simulink model "groundStation001_th"  (R2018b)
settings: Solver=VariableStepAuto  StartTime=0.0  StopTime=sim_time  FixedStep=1e-2  MaxStep=.1  RelTol=1e-3
values from neighbouring files (symbols this model uses):
  initPos = [0 0 100]    [groundStation001_ts.m]    (also in groundStation001_ts2.m)
  objectHeight = platformVolume^(1/3)    (= 1.51829448594)    [groundStation001_ts.m]    (also in groundStation001_ts2.m)
  platformInertiaMatrix = ((1/6)*platformMass*objectHeight^2).*eye(3)    [groundStation001_ts.m]    (also in groundStation001_ts2.m = ((1/6)*platformMass*platformVolume^(2/3)).*eye(3))
  thrs = OCT.tethers    [groundStation001_ts2.m]
libraries: vectorNormalizer_ul x1, constantUniformFlow_ul x1, groundStation001_cl x1
settings Model: Creator=Erin B  LastModifiedBy=Erin B

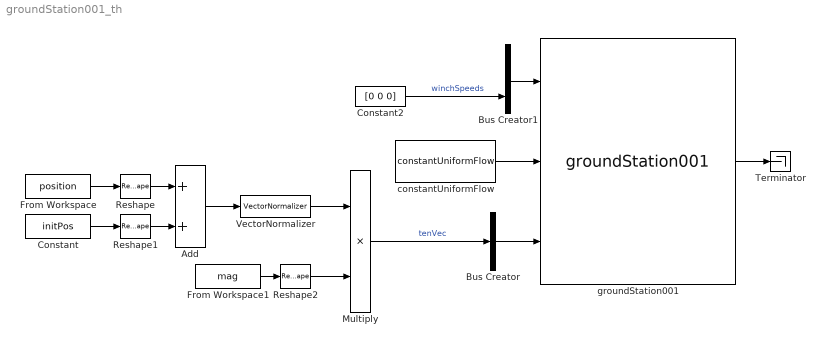
== system groundStation001_th ==
  Add : Sum
  Bus Creator : BusCreator  Inputs=1  OutDataTypeStr=Bus: thrTenVecBus  NonVirtualBus=on
  Bus Creator1 : BusCreator  Inputs=2  OutDataTypeStr=Bus: ctrlBus  NonVirtualBus=on
  Constant : Constant  Value=initPos
  Constant2 : Constant  Value=[0 0 0]
  From Workspace : FromWorkspace  VariableName=position  SampleTime=0
  From Workspace1 : FromWorkspace  VariableName=mag  SampleTime=0
  Multiply : Product
  Reshape : Reshape  OutputDimensionality=Column vector (2-D)
  Reshape1 : Reshape  OutputDimensionality=Column vector (2-D)
  Reshape2 : Reshape  OutputDimensionality=Column vector (2-D)
  Terminator : Terminator
  "VectorNormalizer " : vectorNormalizer_ul/VectorNormalizer   SystemSampleTime=-1
  constantUniformFlow : constantUniformFlow_ul/constantUniformFlow  SystemSampleTime=-1  VariantControl=VSS_environment_constantUniformFlow
  groundStation001 : groundStation001_cl/groundStation001  data=0  moments=1  anchThrPltfrmAttchPts=anchThrPltfrm  anchThrGroundAttchPts=anchThrGnd  airbThrPltfrmAttachPts=airbThrPltfrm  numNodes=thrs.numNodes.Value  thrStructure=thrs.struct('OCT.tether')  tetherLengths=tetherLengths  mass=platformMass  J=platformInertiaMatrix  initPos=initPos  initVel=initVel  initEulAngs=initEulAng  initAngVel=initAngVel  rho=1000  grav=9.81  CM2CBVec=[0 0 objectHeight/4]  vol=platformVolume  h=objectHeight  waveAmplitude=waveAmp  oceanDepth=oceanDepth  wavePeriod=wavePeriod
  wires:
  groundStation001/1 -> Terminator/1
  constantUniformFlow/1 -> groundStation001/2
  Bus Creator/1 -> groundStation001/3
  "VectorNormalizer "/1 -> Multiply/1
  Add/1 -> "VectorNormalizer "/1
  From Workspace/1 -> Reshape/1
  Constant/1 -> Reshape1/1
  From Workspace1/1 -> Reshape2/1
  Multiply/1 -> Bus Creator/1  "tenVec"
  Constant2/1 -> Bus Creator1/2  "winchSpeeds"
  Reshape/1 -> Add/1
  Reshape1/1 -> Add/2
  Reshape2/1 -> Multiply/2
  Bus Creator1/1 -> groundStation001/1
